simulink model "PMSM_Second"  (R2021a)
settings: Solver=VariableStepAuto  StartTime=0.0  StopTime=4  RelTol=1e-3
InitFcn:
  | Ls=7*10^(-3);
  | Lq=Ls;
  | Ld=Ls;
  | 
  | Rs=2.98;
  | Pm=.125;
  | 
  | B=.011*10^(-5);
  | j=.47*10^(-4);
  | 
  | P=2;
libraries: spsControlledVoltageSourceLib x3, spsPermanentMagnetSynchronousMachineLib x1, spsabctodq0Lib x1, spsdq0toabcLib x1, spspowerguiLib x1
settings Model: Creator=User  LastModifiedBy=User
settings SolverCC: AlgebraicLoopSolver=TrustRegion
settings DebuggingCC: SFMachineParentedDataDiag=warning

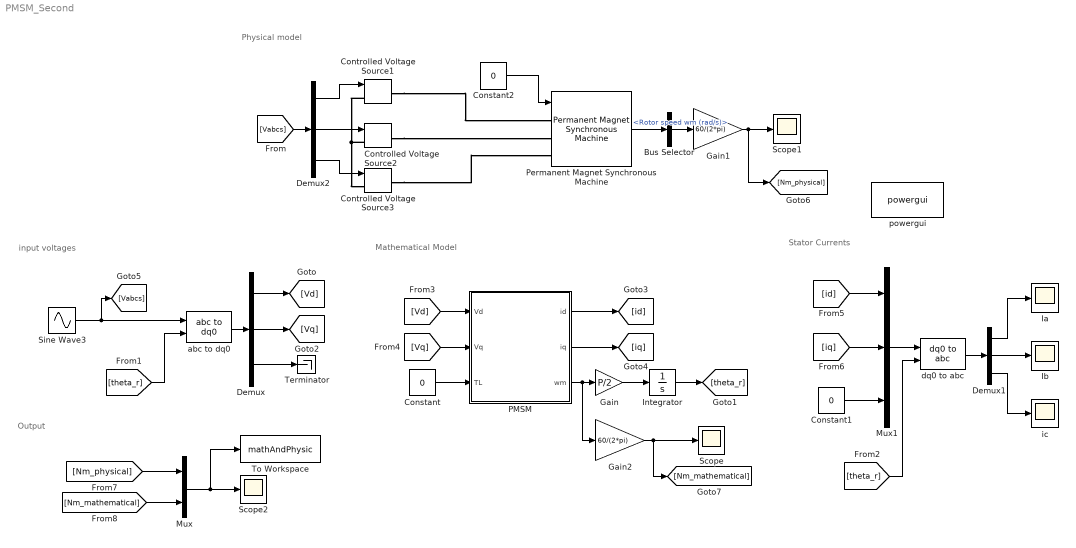
== system PMSM_Second ==
  note: Output
  note: Mathematical Model
  note: Physical model
  note: Stator Currents
  note: input voltages
  Bus Selector : BusSelector  OutputSignals=Rotor speed wm (rad/s)
  Constant : Constant  Value=0
  Constant1 : Constant  Value=0
  Constant2 : Constant  Value=0
  Controlled Voltage Source1 : spsControlledVoltageSourceLib/Controlled Voltage Source  Initialize=on  Source_Type=AC  Amplitude=0  Phase=0  Frequency=0  Measurements=None
  Controlled Voltage Source2 : spsControlledVoltageSourceLib/Controlled Voltage Source  Initialize=on  Source_Type=AC  Amplitude=0  Phase=0  Frequency=0  Measurements=None
  Controlled Voltage Source3 : spsControlledVoltageSourceLib/Controlled Voltage Source  Initialize=on  Source_Type=AC  Amplitude=0  Phase=0  Frequency=0  Measurements=None
  Demux : Demux  Outputs=3
  Demux1 : Demux  Outputs=3
  Demux2 : Demux  Outputs=3
  Gain : Gain  Gain=P/2
  Gain1 : Gain  Gain=60/(2*pi)
  Gain2 : Gain  Gain=60/(2*pi)
  Ia : Scope
  Ib : Scope
  Integrator : Integrator
  Mux : Mux  Inputs=2
  Mux1 : Mux  Inputs=3
  PMSM : Subsystem
  Permanent Magnet Synchronous Machine : spsPermanentMagnetSynchronousMachineLib/Permanent Magnet Synchronous Machine  NbPhases=3  FluxDistribution=Sinusoidal  RotorType=Round  MechanicalLoad=Torque Tm  PresetModel=No  ShowDetailedParameters=on  MeasurementBus=off  Resistance=Rs  Inductance=8.5e-3  dqInductances=[8.5e-3,8.5e-3]  La=Ls  MachineConstant=Flux linkage established by magnets (V.s)  Flux=Pm  VoltageCst=51.8307  TorqueCst=0.42864  Flat=120  Mechanical=[j B P/2 0]  PolePairs=4  InitialConditions=[0,0, 0,0]  InitialConditions5ph=[0 0 0 0 0 0]  RefAngle=Aligned with phase A axis (original Park)  IterativeDiscreteModel=Trapezoidal non iterative  TsBlock=-1  TsPowergui=0
  Scope : Scope
  Scope1 : Scope
  Scope2 : Scope
  Sine Wave3 : Sin  Amplitude=220*sqrt(2)  Frequency=2*pi*50  Phase=[0 -2*pi/3 2*pi/3]  SampleTime=0
  Terminator : Terminator
  To Workspace : ToWorkspace  VariableName=mathAndPhysic  SaveFormat=Timeseries  SampleTime=-1
  abc to dq0 : spsabctodq0Lib/abc to dq0  Alignment=Aligned with phase A axis
  dq0 to abc : spsdq0toabcLib/dq0 to abc  Alignment=Aligned with phase A axis
  ic : Scope
  powergui : spspowerguiLib/powergui  Priority=1  SimulationMode=Continuous  SampleTime=50e-6  frequency=60  Iterations=50  frequencyindice=0  Pbase=100e6  ErrMax=1e-4  UnitsV=kV  UnitsW=MW  buscounter=0  FunctionMessages=off  echomessages=off  EnableUseOfTLC=off  CurrentSourceSwitches=off  DisableSnubberDevices=on  DisableRonSwitches=on  DisableVfSwitches=on  DisplayEquations=off  AutomaticDiscreteSolvers=off  SolverType=Tustin/Backward Euler (TBE)  Interpol=off  ExternalGateDelay=off  methode=off  Ts=100  x0status=blocks  SPID=on  SwTol=0  HookPort=off  NonlinearTolerance=1e-4  nMaxIteration=100  ContinueOnMaxIteration=off  RestoreLinks=warning  ResistiveCurrentMeasurement=off  Frange=[0:2:500]  Ylog=off  Xlog=on  ShowGrid=off  save=off  variable=ZData  structure=0  ZoomFFT=off  StartTime=0.0  cycles=1  DisplayStyle=1  fundamental=60  FreqAxis=off  MaxFrequency=1000  frequencyindicesteady=1  RmsSteady=1  display=off
  wires:
  Sine Wave3/1 -> [Vabcs], abc to dq0/1
  abc to dq0/1 -> Demux/1
  Demux/3 -> Terminator/1
  Mux1/1 -> dq0 to abc/1
  Constant1/1 -> Mux1/3
  Integrator/1 -> [theta_r]
  [theta_r] -> abc to dq0/2
  [theta_r] -> dq0 to abc/2
  dq0 to abc/1 -> Demux1/1
  PMSM/3(wm) -> Gain2/1, Gain/1
  Gain/1 -> Integrator/1
  Demux/1 -> [Vd]
  Demux/2 -> [Vq]
  [Vd] -> PMSM/1(Vd)
  [Vq] -> PMSM/2(Vq)
  Constant/1 -> PMSM/3(TL)
  PMSM/1(id) -> [id]
  PMSM/2(iq) -> [iq]
  [id] -> Mux1/1
  [iq] -> Mux1/2
  Demux1/1 -> Ia/1
  Demux1/2 -> Ib/1
  Demux1/3 -> ic/1
  Constant2/1 -> Permanent Magnet Synchronous Machine/1
  Permanent Magnet Synchronous Machine/1 -> Bus Selector/1
  Gain1/1 -> [Nm_physical], Scope1/1
  Bus Selector/1 -> Gain1/1  "<Rotor speed wm (rad/s)>"
  Gain2/1 -> [Nm_mathematical], Scope/1
  [Vabcs] -> Demux2/1
  Demux2/1 -> Controlled Voltage Source1/1
  Demux2/2 -> Controlled Voltage Source2/1
  Demux2/3 -> Controlled Voltage Source3/1
  [Nm_physical] -> Mux/1
  [Nm_mathematical] -> Mux/2
  Mux/1 -> To Workspace/1, Scope2/1
  connections:
  Controlled Voltage Source1/RConn1 -- Permanent Magnet Synchronous Machine/LConn1
  Controlled Voltage Source2/RConn1 -- Permanent Magnet Synchronous Machine/LConn2
  Controlled Voltage Source3/RConn1 -- Permanent Magnet Synchronous Machine/LConn3
  Controlled Voltage Source1/LConn1 -- Controlled Voltage Source3/LConn1 -- Controlled Voltage Source2/LConn1

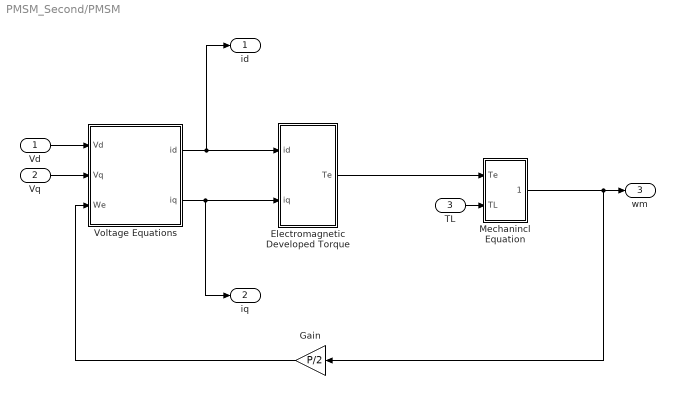
== system PMSM_Second/PMSM ==
  Vd : Inport
  Vq : Inport  Port=2
  TL : Inport  Port=3
  Electromagnetic Developed Torque : Subsystem
  Gain : Gain  Gain=P/2
  Mechanincl Equation : Subsystem
  Voltage Equations : Subsystem
  id : Outport
  iq : Outport  Port=2
  wm : Outport  Port=3
  wires:
  Vd/1 -> Voltage Equations/1(Vd)
  Voltage Equations/1(id) -> Electromagnetic Developed Torque/1(id), id/1
  Mechanincl Equation/1(wm) -> Gain/1, wm/1
  Voltage Equations/2(iq) -> Electromagnetic Developed Torque/2(iq), iq/1
  Electromagnetic Developed Torque/1(Te) -> Mechanincl Equation/1(Te)
  Vq/1 -> Voltage Equations/2(Vq)
  TL/1 -> Mechanincl Equation/2(TL)
  Gain/1 -> Voltage Equations/3(We)

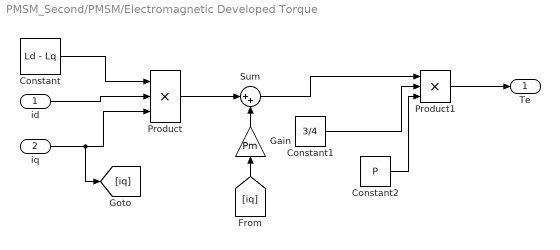
== system PMSM_Second/PMSM/Electromagnetic Developed Torque ==
  id : Inport
  iq : Inport  Port=2
  Constant : Constant  Value=Ld - Lq
  Constant1 : Constant  Value=3/4
  Constant2 : Constant  Value=P
  Gain : Gain  Gain=Pm
  Product : Product  Inputs=3
  Product1 : Product  Inputs=3
  Sum : Sum  Inputs=|++
  Te : Outport
  wires:
  Sum/1 -> Product1/1
  Product/1 -> Sum/1
  id/1 -> Product/2
  iq/1 -> [iq], Product/3
  Product1/1 -> Te/1
  Constant1/1 -> Product1/2
  Constant2/1 -> Product1/3
  Constant/1 -> Product/1
  Gain/1 -> Sum/2
  [iq] -> Gain/1

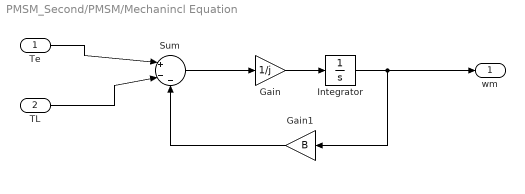
== system PMSM_Second/PMSM/Mechanincl Equation ==
  Te : Inport
  TL : Inport  Port=2
  Gain : Gain  Gain=1/j
  Gain1 : Gain  Gain=B
  Integrator : Integrator
  Sum : Sum  Inputs=|+--
  wm : Outport
  wires:
  Gain/1 -> Integrator/1
  Te/1 -> Sum/1
  Gain1/1 -> Sum/3
  Integrator/1 -> wm/1, Gain1/1
  TL/1 -> Sum/2
  Sum/1 -> Gain/1

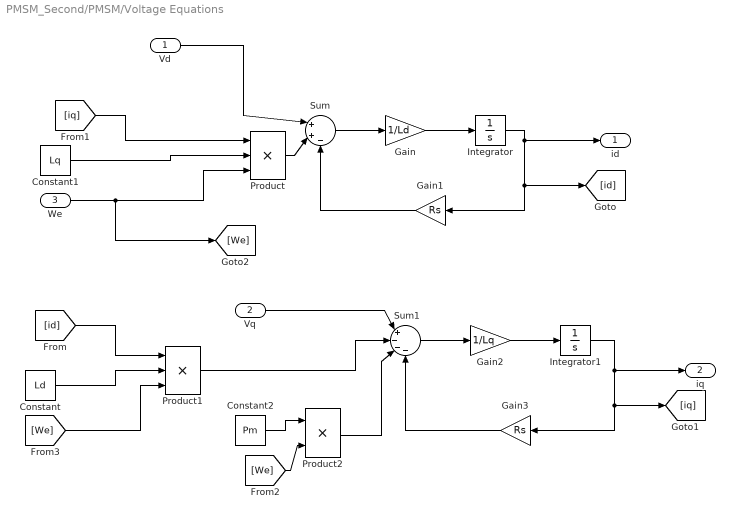
== system PMSM_Second/PMSM/Voltage Equations ==
  Vd : Inport
  Vq : Inport  Port=2
  We : Inport  Port=3
  Constant : Constant  Value=Ld
  Constant1 : Constant  Value=Lq
  Constant2 : Constant  Value=Pm
  Gain : Gain  Gain=1/Ld
  Gain1 : Gain  Gain=Rs
  Gain2 : Gain  Gain=1/Lq
  Gain3 : Gain  Gain=Rs
  Integrator : Integrator
  Integrator1 : Integrator
  Product : Product  Inputs=3
  Product1 : Product  Inputs=3
  Product2 : Product
  Sum : Sum  Inputs=|++-
  Sum1 : Sum  Inputs=|+---
  id : Outport
  iq : Outport  Port=2
  wires:
  Integrator/1 -> id/1, Gain1/1, [id]
  [iq] -> Product/1
  Constant2/1 -> Product2/1
  We/1 -> [We], Product/3
  Product/1 -> Sum/2
  Integrator1/1 -> iq/1, [iq], Gain3/1
  Vq/1 -> Sum1/1
  Gain/1 -> Integrator/1
  Constant1/1 -> Product/2
  Product2/1 -> Sum1/3
  Sum/1 -> Gain/1
  Constant/1 -> Product1/2
  [We] -> Product2/2
  Gain3/1 -> Sum1/4
  Gain2/1 -> Integrator1/1
  Sum1/1 -> Gain2/1
  Vd/1 -> Sum/1
  Gain1/1 -> Sum/3
  [id] -> Product1/1
  Product1/1 -> Sum1/2
  [We] -> Product1/3
